simulink library "xbsStateMachine"  (Simulink 4.00)
undefined symbols (not defined in the file or in its folder): xlDistRamDepth, xlMatrixToOutputVec, xlMatrixToStateInitVec, xlNumMealyElements, xlNumMooreOutputElements, xlNumMooreStateElements, xlNumStateBits, xlRegMealyInitVec
libraries: xbsMemory x7, xbsBasic x6
settings Model: Creator=Administrator  LastModifiedBy=haibing

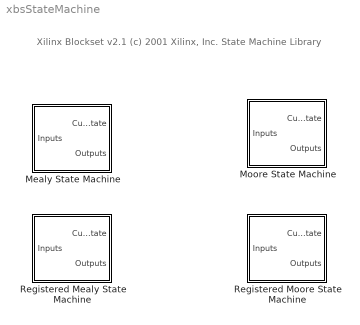
== system xbsStateMachine ==
  note: Xilinx Blockset v2.1
      | (c) 2001 Xilinx, Inc.
      |
      | State Machine Library
  Mealy State Machine : Subsystem  mask(Mealy State Machine){next_state_matrix=[0 1; 2 1; 0 3; 2 1], output_matrix=[0 0; 0 0; 0 0; 0 1], n_bits=1, period=1}
      mask prompts: next_state_matrix "Next State Matrix"; output_matrix "Output Matrix"; n_bits "Number of  Output Bits"; period "Sample Period"
      mask help: The output of this state machine is a function of the current state and its input.
      mask init:
      | % Set Block Logo
      | [bg,fg] = xlcmap('XBlock',0);
      | iPos = get_param(gcb,'Position');
      | iWidth=iPos(3)-iPos(1); iHeight=iPos(4)-iPos(2);
      | iCx=iWidth/2;
      | iCy=iHeight/2;
      | [logoX, logoY] = xlogo(iPos);
      settings: RTWFcnNameOpts=Auto  RTWFileNameOpts=Auto
      mask Help: web(xldoclink('Mealy State Machine'));
      mask Display:
      | patch([0 iWidth iWidth 0],[0 0 iHeight iHeight] , bg);
      | patch(logoX,logoY, fg);
      | port_label('input',1,'Inputs');
      | port_label('output',1,'CurrentState');
      | port_label('output',2,'Outputs');
      | 
      | plot([0 0 iWidth iWidth 0], [0 iHeight iHeight 0 0]);
  Moore State Machine : Subsystem  mask(Moore State Machine){next_state_matrix=[0 1; 2 1; 0 3; 2 4; 0 1], output_matrix=[0; 0; 0; 0; 1], n_bits=1, period=1}
      mask prompts: next_state_matrix "Next State Matrix"; output_matrix "Output Array"; n_bits "Number of Output Bits"; period "Sample Period"
      mask help: The output of this state machine is a function of only the current state.
      mask init:
      | % Set Block Logo
      | [bg,fg] = xlcmap('XBlock',0);
      | iPos = get_param(gcb,'Position');
      | iWidth=iPos(3)-iPos(1); iHeight=iPos(4)-iPos(2);
      | iCx=iWidth/2;
      | iCy=iHeight/2;
      | [logoX, logoY] = xlogo(iPos);
      settings: RTWFcnNameOpts=Auto  RTWFileNameOpts=Auto
      mask Help: web(xldoclink('Moore State Machine'));
      mask Display:
      | patch([0 iWidth iWidth 0],[0 0 iHeight iHeight] , bg);
      | patch(logoX,logoY, fg);
      | port_label('input',1,'Inputs');
      | port_label('output',1,'CurrentState');
      | port_label('output',2,'Outputs');
      | 
      | plot([0 0 iWidth iWidth 0], [0 iHeight iHeight 0 0]);
  Registered Mealy State Machine : Subsystem  mask(Registered Mealy State Machine){next_state_matrix=[0 1; 2 1; 0 3; 2 1], output_matrix=[0 0; 0 0; 0 0; 0 1], n_bits=1, period=1}
      mask prompts: next_state_matrix "Next State Matrix"; output_matrix "Output Matrix"; n_bits "Number of Output Bits"; period "Sample Period"
      mask help: The output of this state machine is a function of the current state and its input. The output of the state machine is registered.
      mask init:
      | % Set Block Logo
      | [bg,fg] = xlcmap('XBlock',0);
      | iPos = get_param(gcb,'Position');
      | iWidth=iPos(3)-iPos(1); iHeight=iPos(4)-iPos(2);
      | iCx=iWidth/2;
      | iCy=iHeight/2;
      | [logoX, logoY] = xlogo(iPos);
      settings: RTWFcnNameOpts=Auto  RTWFileNameOpts=Auto
      mask Help: web(xldoclink('Registered Mealy State Machine'));
      mask Display:
      | patch([0 iWidth iWidth 0],[0 0 iHeight iHeight] , bg);
      | patch(logoX,logoY, fg);
      | port_label('input',1,'Inputs');
      | port_label('output',1,'CurrentState');
      | port_label('output',2,'Outputs');
      | 
      | plot([0 0 iWidth iWidth 0], [0 iHeight iHeight 0 0]);
  Registered Moore State Machine : Subsystem  mask(Moore State Machine){next_state_matrix=[0 1; 2 1; 0 3; 2 4; 0 1], output_matrix=[0; 0; 0; 0; 1], n_bits=1, period=1}
      mask prompts: next_state_matrix "Next State Matrix"; output_matrix "Output Array"; n_bits "Number of Output Bits"; period "Sample Period"
      mask help: The output of this state machine is a function of only the current state. The output of the state machine is registered.
      mask init:
      | % Set Block Logo
      | [bg,fg] = xlcmap('XBlock',0);
      | iPos = get_param(gcb,'Position');
      | iWidth=iPos(3)-iPos(1); iHeight=iPos(4)-iPos(2);
      | iCx=iWidth/2;
      | iCy=iHeight/2;
      | [logoX, logoY] = xlogo(iPos);
      settings: RTWFcnNameOpts=Auto  RTWFileNameOpts=Auto
      mask Help: web(xldoclink('Registered Moore State Machine'));
      mask Display:
      | patch([0 iWidth iWidth 0],[0 0 iHeight iHeight] , bg);
      | patch(logoX,logoY, fg);
      | port_label('input',1,'Inputs');
      | port_label('output',1,'CurrentState');
      | port_label('output',2,'Outputs');
      | 
      | plot([0 0 iWidth iWidth 0], [0 iHeight iHeight 0 0]);

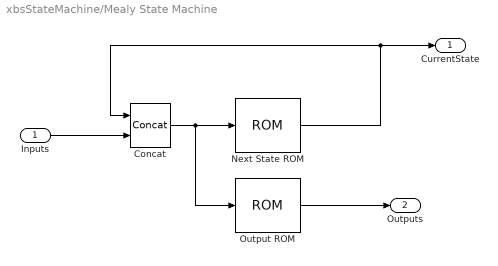
== system xbsStateMachine/Mealy State Machine ==
  Inputs : Inport  Port=1
  Concat : xbsBasic/Concat  explicit_period=off  period=1  dbl_ovrd=off  version=1.1
  Next State ROM : xbsMemory/ROM  depth=xlNumMealyElements(next_state_matrix, output_matrix)  initVector=xlMatrixToStateInitVec(next_state_matrix,xlNumStateBits(next_state_matrix),0,1,1,1)  arith_type=Unsigned  n_bits=xlNumStateBits(next_state_matrix)  bin_pt=0  quantization=Truncate  overflow=Wrap  latency=1  explicit_period=on  period=period  init_zero=on  dbl_ovrd=off  distributed_mem=off  gen_core=on  version=1.1
  Output ROM : xbsMemory/ROM  depth=xlDistRamDepth(output_matrix)  initVector=xlMatrixToOutputVec(output_matrix,n_bits,0,1,1,1)  arith_type=Unsigned  n_bits=n_bits  bin_pt=0  quantization=Truncate  overflow=Wrap  latency=0  explicit_period=on  period=period  init_zero=on  dbl_ovrd=off  distributed_mem=on  gen_core=on  version=1.1
  CurrentState : Outport  Port=1
  Outputs : Outport  Port=2
  wires:
  Inputs/1 -> Concat/2
  Output ROM/1 -> Outputs/1
  Concat/1 -> Next State ROM/1, Output ROM/1
  Next State ROM/1 -> Concat/1, CurrentState/1

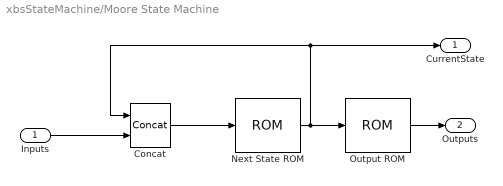
== system xbsStateMachine/Moore State Machine ==
  Inputs : Inport  Port=1
  Concat : xbsBasic/Concat  explicit_period=off  period=1  dbl_ovrd=off  version=1.1
  Next State ROM : xbsMemory/ROM  depth=xlNumMooreStateElements(next_state_matrix, output_matrix)  initVector=xlMatrixToStateInitVec(next_state_matrix,xlNumStateBits(next_state_matrix),0,1,1,1)  arith_type=Unsigned  n_bits=xlNumStateBits(next_state_matrix)  bin_pt=0  quantization=Truncate  overflow=Wrap  latency=1  explicit_period=on  period=period  init_zero=on  dbl_ovrd=off  distributed_mem=off  gen_core=on  version=1.1
  Output ROM : xbsMemory/ROM  depth=xlDistRamDepth(output_matrix)  initVector=xlMatrixToOutputVec(output_matrix,n_bits,0,1,1,1)  arith_type=Unsigned  n_bits=n_bits  bin_pt=0  quantization=Truncate  overflow=Wrap  latency=0  explicit_period=on  period=period  init_zero=on  dbl_ovrd=off  distributed_mem=on  gen_core=on  version=1.1
  CurrentState : Outport  Port=1
  Outputs : Outport  Port=2
  wires:
  Inputs/1 -> Concat/2
  Output ROM/1 -> Outputs/1
  Concat/1 -> Next State ROM/1
  Next State ROM/1 -> Concat/1, CurrentState/1, Output ROM/1

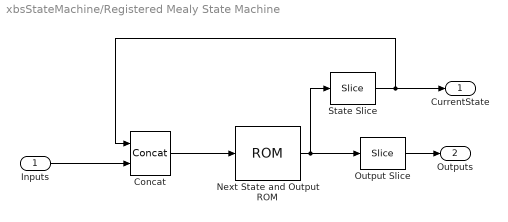
== system xbsStateMachine/Registered Mealy State Machine ==
  Inputs : Inport  Port=1
  Concat : xbsBasic/Concat  explicit_period=off  period=1  dbl_ovrd=off  version=1.1
  Next State and Output ROM : xbsMemory/ROM  depth=xlNumMealyElements(next_state_matrix, output_matrix)  initVector=xlRegMealyInitVec(next_state_matrix, output_matrix, n_bits,0,1,1,1)  arith_type=Unsigned  n_bits=xlNumStateBits(next_state_matrix)+n_bits  bin_pt=0  quantization=Truncate  overflow=Wrap  latency=1  explicit_period=on  period=period  init_zero=on  dbl_ovrd=off  distributed_mem=off  gen_core=on  version=1.1
  Output Slice : xbsBasic/Slice  mode=Lower Bit Location + Width  nbits=n_bits  bit1=0  base1=MSB of Input  bit0=0  base0=LSB of Input  explicit_period=off  period=1  dbl_ovrd=off  version=1.1
  State Slice : xbsBasic/Slice  mode=Upper Bit Location + Width  nbits=xlNumStateBits(next_state_matrix)  bit1=0  base1=MSB of Input  bit0=0  base0=LSB of Input  explicit_period=off  period=1  dbl_ovrd=off  version=1.1
  CurrentState : Outport  Port=1
  Outputs : Outport  Port=2
  wires:
  Inputs/1 -> Concat/2
  Output Slice/1 -> Outputs/1
  Concat/1 -> Next State and Output ROM/1
  Next State and Output ROM/1 -> Output Slice/1, State Slice/1
  State Slice/1 -> CurrentState/1, Concat/1

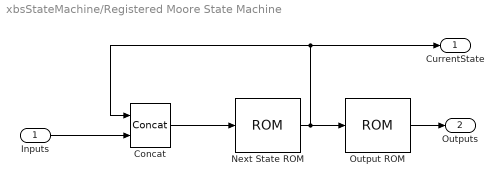
== system xbsStateMachine/Registered Moore State Machine ==
  Inputs : Inport  Port=1
  Concat : xbsBasic/Concat  explicit_period=off  period=1  dbl_ovrd=off  version=1.1
  Next State ROM : xbsMemory/ROM  depth=xlNumMooreStateElements(next_state_matrix, output_matrix)  initVector=xlMatrixToStateInitVec(next_state_matrix,xlNumStateBits(next_state_matrix),0,1,1,1)  arith_type=Unsigned  n_bits=xlNumStateBits(next_state_matrix)  bin_pt=0  quantization=Truncate  overflow=Wrap  latency=1  explicit_period=on  period=period  init_zero=on  dbl_ovrd=off  distributed_mem=off  gen_core=on  version=1.1
  Output ROM : xbsMemory/ROM  depth=xlNumMooreOutputElements(output_matrix)  initVector=xlMatrixToOutputVec(output_matrix,n_bits,0,1,1,1)  arith_type=Unsigned  n_bits=n_bits  bin_pt=0  quantization=Truncate  overflow=Wrap  latency=1  explicit_period=on  period=period  init_zero=on  dbl_ovrd=off  distributed_mem=off  gen_core=on  version=1.1
  CurrentState : Outport  Port=1
  Outputs : Outport  Port=2
  wires:
  Next State ROM/1 -> Output ROM/1, CurrentState/1, Concat/1
  Concat/1 -> Next State ROM/1
  Output ROM/1 -> Outputs/1
  Inputs/1 -> Concat/2
